simulink model "FaultCheck"  (R2022b)
settings: Solver=FixedStepAuto  StartTime=0.0  StopTime=10  FixedStep=1  RelTol=1e-3
undefined symbols (not defined in the file): C_Flt_IGBTULowerTempConfirmTh_u16, C_Flt_IGBTULowerTempDiagEn_b, C_Flt_IGBTULowerTempErrCode_u16, C_Flt_IGBTULowerTempPowerCoeff, C_Flt_IGBTULowerTempRecoveryTh_u16, C_Flt_IGBTULowerTempRecTh_s32, C_Flt_IGBTULowerTempTrigTh_s32, C_Flt_IGBTUOverTempConfirmTh_u16, C_Flt_IGBTUOverTempDiagEn_b, C_Flt_IGBTUOverTempErrCode_u16, C_Flt_IGBTUOverTempRecoveryTh_u16, C_Flt_IGBTUOverTempRecTh_s32, C_Flt_IGBTUOverTempTrigTh_s32, C_Flt_IGBTVLowerTempConfirmTh_u16, C_Flt_IGBTVLowerTempDiagEn_b, C_Flt_IGBTVLowerTempErrCode_u16, C_Flt_IGBTVLowerTempPowerCoeff, C_Flt_IGBTVLowerTempRecoveryTh_u16, C_Flt_IGBTVLowerTempRecTh_s32, C_Flt_IGBTVLowerTempTrigTh_s32, C_Flt_IGBTVOverTempConfirmTh_u16, C_Flt_IGBTVOverTempDiagEn_b, C_Flt_IGBTVOverTempErrCode_u16, C_Flt_IGBTVOverTempRecoveryTh_u16, C_Flt_IGBTVOverTempRecTh_s32, C_Flt_IGBTVOverTempTrigTh_s32, C_Flt_IGBTWLowerTempConfirmTh_u16, C_Flt_IGBTWLowerTempDiagEn_b, C_Flt_IGBTWLowerTempErrCode_u16, C_Flt_IGBTWLowerTempPowerCoeff, C_Flt_IGBTWLowerTempRecoveryTh_u16, C_Flt_IGBTWLowerTempRecTh_s32, C_Flt_IGBTWLowerTempTrigTh_s32, C_Flt_IGBTWOverTempConfirmTh_u16, C_Flt_IGBTWOverTempDiagEn_b, C_Flt_IGBTWOverTempErrCode_u16, C_Flt_IGBTWOverTempRecoveryTh_u16, C_Flt_IGBTWOverTempRecTh_s32, C_Flt_IGBTWOverTempTrigTh_s32, C_Flt_IuOCConfirmTh_u16, C_Flt_IuOCDiagEn_b, C_Flt_IuOCErrCode_u16, C_Flt_IuOCNegLimit_s32, C_Flt_IuOCPosLimit_s32, C_Flt_IuOCRecoveryTh_u16, C_Flt_IuZeroDriftDiagEn_b, C_Flt_IuZeroDriftErrCode_u16, C_Flt_IvOCConfirmTh_u16, C_Flt_IvOCDiagEn_b, C_Flt_IvOCErrCode_u16, C_Flt_IvOCNegLimit_s32, C_Flt_IvOCPosLimit_s32, C_Flt_IvOCRecoveryTh_u16, C_Flt_IvZeroDriftDiagEn_b, C_Flt_IvZeroDriftErrCode_u16, C_Flt_IwOCConfirmTh_u16, C_Flt_IwOCDiagEn_b, C_Flt_IwOCErrCode_u16, C_Flt_IwOCNegLimit_s32, C_Flt_IwOCPosLimit_s32 ... (+196)
libraries: YS_UserDefined_Library x21, simulink x5
(part 2 of 11)

== system FaultCheck/FaultDiag_HighTask_100us/FltDetn/RecUDetn ==
  note: Flt_RecU_ErrDeb
      | Uint8
      | 旋变电压故障判断次数
      |
      | Flt_RecU_ActvnErrDetn
      | Uint8
      | 旋变电压故障使能标志位
      |
      | Flt_RecU_ErrCode
      | Uint16
      | 旋变电压故障码
  note: 故障诊断主体模块主要包括四个部分，故障诊断标志位判断、故障等级判断、降功率系数判断和故障码记录
      | 1、故障诊断标志位判断：根据使能标志位判断进入，最后确认其故障标志位的值
      | 2、故障码记录：根据故障标志位记录相关故障码，0还是标定量。
      | 3、故障等级判断：根据故障标志位确定相关故障等级，是0还是标定量
      | 4、降功率系数判断：根据故障等级进行判断选择对应的降功率系数
      |
      | 故障标志位的判断：
      | 当输入的旋变供电标志位标志位为1，并持续标定的次数，故障标志位置1，否者保留上一时刻的故障标志位0，不可恢复。
  IPT_Res_Udc_Error_Flg : Inport
  Sys_SelfChkFishFlg : Inport  Port=2
  Bus Creator : BusCreator  Inputs=2
  Enable : Subsystem
  Parameter : Subsystem
  RecUDetn : Subsystem
  Flt_RecUDetnOut : Outport
  wires:
  Sys_SelfChkFishFlg/1 -> Enable/1(Sys_SelfChkFishFlg)
  Enable/1(Enable) -> RecUDetn/2(EnabDetn)
  RecUDetn/1(Flt_RecUFltLvl) -> Bus Creator/1
  RecUDetn/2(Flt_RecUPowRecCoefOut) -> Bus Creator/2
  Parameter/1(Para) -> RecUDetn/3(Para)
  Bus Creator/1 -> Flt_RecUDetnOut/1
  IPT_Res_Udc_Error_Flg/1 -> RecUDetn/1(InPutVal)

== system FaultCheck/FaultDiag_HighTask_100us/FltDetn/ResErrFlgDetn ==
  note: Flt_ResErr_ActvnDetn
      | Uint8
      | 旋变信号故障判断次数
      |
      | Flt_ResErr_ErrCode
      | Uint16
      | 旋变信号故障码
  note: 故障诊断主体模块主要包括四个部分，故障诊断标志位判断、故障等级判断、降功率系数判断和故障码记录
      | 1、故障诊断标志位判断：根据使能标志位判断进入，最后确认其故障标志位的值
      | 2、故障码记录：根据故障标志位记录相关故障码，0还是标定量。
      | 3、故障等级判断：根据故障标志位确定相关故障等级，是0还是标定量
      | 4、降功率系数判断：根据故障等级进行判断选择对应的降功率系数
      |
      | 故障标志位的判断：
      | 当输入的旋变信号故障标志位标志位为1，并持续标定的次数，故障标志位置1，否者保留上一时刻的故障标志位0，不可恢复。
  IPT_Hw_RES_LOT_Error_Flg : Inport
  IPT_Hw_RES_LOS_Error_Flg : Inport  Port=2
  Sys_SelfChkFishFlg : Inport  Port=3
  Bus Creator : BusCreator  Inputs=2
  Enable : Subsystem
  Logical Operator : Logic  Operator=OR  AllPortsSameDT=off  OutDataTypeStr=boolean
  Parameter : Subsystem
  ResErrDetn : Subsystem
  Flt_ResErrFlgDetnOut : Outport
  wires:
  Enable/1(Enable) -> ResErrDetn/2(EnabDetn)
  ResErrDetn/1(Flt_ResErrFltLvl) -> Bus Creator/1
  ResErrDetn/2(Flt_ResErrPowRecCoefOut) -> Bus Creator/2
  Parameter/1(Para) -> ResErrDetn/3(Para)
  Bus Creator/1 -> Flt_ResErrFlgDetnOut/1
  Sys_SelfChkFishFlg/1 -> Enable/1(Sys_SelfChkFishFlg)
  IPT_Hw_RES_LOT_Error_Flg/1 -> Logical Operator/1
  IPT_Hw_RES_LOS_Error_Flg/1 -> Logical Operator/2
  Logical Operator/1 -> ResErrDetn/1(InPutVal1)

== system FaultCheck/FaultDiag_HighTask_100us/FltDetn/ResolveSensorDetn ==
  Sys_SelfChkFishFlg : Inport
  Flt_ResolveSensorFlg : Inport  Port=2
  Bus Creator : BusCreator  Inputs=2
  Enable : Subsystem
  Flt_ResolveSensorDetn : Subsystem
  Parameter : Subsystem
  Flt_ResolveSensorDetnOut : Outport
  wires:
  Parameter/1(Para) -> Flt_ResolveSensorDetn/3(Para)
  Enable/1(Enable) -> Flt_ResolveSensorDetn/2(EnabDetn)
  Bus Creator/1 -> Flt_ResolveSensorDetnOut/1
  Sys_SelfChkFishFlg/1 -> Enable/1(Sys_SelfChkFishFlg)
  Flt_ResolveSensorDetn/2(Flt_ResolveSensorPowRecCoefOut) -> Bus Creator/2
  Flt_ResolveSensorDetn/1(Flt_ResolveSensorFltLvl) -> Bus Creator/1
  Flt_ResolveSensorFlg/1 -> Flt_ResolveSensorDetn/1(InPutVal1)

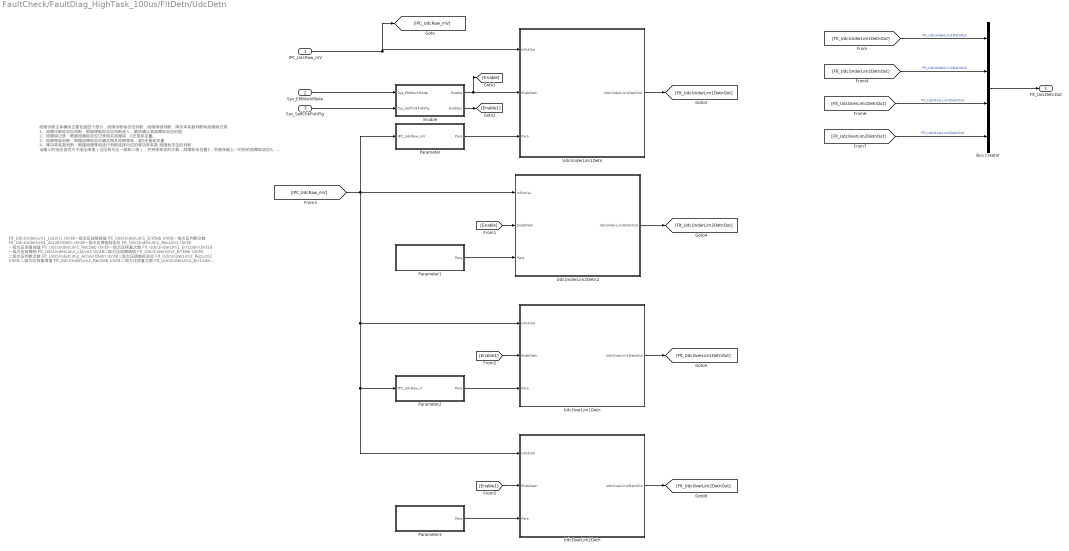
== system FaultCheck/FaultDiag_HighTask_100us/FltDetn/UdcDetn ==
  note: Flt_UdcUnderLim1_LoLim1
      | Uint8
      | 一级欠压故障阈值
      |
      | Flt_UdcUnderLim1_ErrDeb
      | Uint8
      | 一级欠压判断次数
      |
      | Flt_UdcUnderLim1_ActvErrDetn
      | Uint8
      | 一级欠压使能标志位
      |
      | Flt_UdcUnderLim1_RecLim1
      | Uint8
      | 一级欠压恢复阈值
      |
      | Flt_UdcUnderLim1_RecDeb
      | Uint8
      | 一级欠压恢复次数
      |
      | Flt_UdcUnderLim1_ErrCode
      | Uint16
      | 一级欠压故障码
      |
      | Flt_UdcUnderLim2_LoLim2
      | Uint8
      | 二级欠压故障阈值
      |
      | Flt_UdcUnderLim2_ErrDeb
      | Uint8
      | 二级欠压判断次数
      |
      | Flt_UdcUnderLim2_ActvErrDetn
      | Uint8
      | 二级欠压使能标志位
      |
      | Flt_UdcUnderLim2_RecLim2
      | Uint8
      | 二级欠压恢复阈值
      |
      | Flt_UdcUnderLim2_RecDeb
      | Uint8
      | 二级欠压恢复次数
      |
      | Flt_UdcUnderLim2_ErrCode
      | Uint16
      | 二级欠压故障码
      |
      | Flt_UdcOverLim1_OverLim1
      | Uint8
      | 一级过压故障阈值
      |
      | Flt_UdcOverLim1_ErrDeb
      | Uint8
      | 一级过压判断次数
      |
      | Flt_UdcOverLim1_ActvErrDetn
      | Uint8
      | 一级过压使能标志位
      |
      | Flt_UdcOverLim1_RecLim1
      | Uint8
      | 一级过压恢复阈值
      |
      | Flt_UdcOverLim1_RecDeb
      | Uint8
      | 一级过压恢复次数
      |
      | Flt_UdcOverLim1_ErrCode
      | Uint16
      | 一级过压故障码
      |
      | Flt_UdcOverLim2_OverLim2
      | Uint8
      | 二过压故障阈值
      |
      | Flt_UdcOverLim2_ErrDeb
      | Uint8
      | 二级过压判断次数
      |
      | Flt_UdcOverLim2_ActvErrDetn
      | Uint8
      | 二级过压使能标志位
      |
      | Flt_UdcOverLim2_ErrCode
      | Uint16
      | 二级过压故障码
  note: 故障诊断主体模块主要包括四个部分，故障诊断标志位判断、故障等级判断、降功率系数判断和故障码记录
      | 1、故障诊断标志位判断：根据使能标志位判断进入，最后确认其故障标志位的值
      | 2、故障码记录：根据故障标志位记录相关故障码，0还是标定量。
      | 3、故障等级判断：根据故障标志位确定相关故障等级，是0还是标定量
      | 4、降功率系数判断：根据故障等级进行判断选择对应的降功率系数
      |
      | 故障标志位的判断：
      | 当输入的电压信号大于电压阈值（过压和欠压一级和二级），并持续标定的次数，故障标志位置1，否者保留上一时刻的故障标志位0。
      |
      | 一级和二级欠压，一级过压可恢复，即当输入的电压信号小于恢复的阈值并持续标定的次数，故障标志位置0
      |
      | 二级过压不可恢复
  IPC_UdcRaw_mV : Inport
  Sys_EMWorkMode : Inport  Port=2
  Sys_SelfChkFishFlg : Inport  Port=3
  Bus Creator : BusCreator  Inputs=4
  Enable : Subsystem
  Parameter : Subsystem
  Parameter1 : Subsystem
  Parameter2 : Subsystem
  Parameter3 : Subsystem
  UdcOverLim1Detn : Subsystem
  UdcOverLim2Detn : Subsystem
  UdcUnderLim1Detn : Subsystem
  UdcUnderLim2Detn2 : Subsystem
  Flt_UdcDetnOut : Outport
  wires:
  [IPC_UdcRaw_mV] -> UdcUnderLim2Detn2/1(InPutVal), Parameter/1(IPC_UdcRaw_mV), UdcOverLim2Detn/1(InPutVal), Parameter2/1(IPC_UdcRaw_V), UdcOverLim1Detn/1(InPutVal)
  [Flt_UdcOverLim2DetnOut] -> Bus Creator/4  "Flt_UdcOverLim2DetnOut"
  [Flt_UdcOverLim1DetnOut] -> Bus Creator/3  "Flt_UdcOverLim1DetnOut"
  [Flt_UdcUnderLim2DetnOut] -> Bus Creator/2  "Flt_UdcUnderLim2DetnOut"
  [Flt_UdcUnderLim1DetnOut] -> Bus Creator/1  "Flt_UdcUnderLim1DetnOut"
  UdcOverLim2Detn/1(UdcOverLim2DetnOut) -> [Flt_UdcOverLim2DetnOut]
  UdcOverLim1Detn/1(UdcOverLim1DetnOut) -> [Flt_UdcOverLim1DetnOut]
  UdcUnderLim2Detn2/1(UdcUnderLim2DetnOut) -> [Flt_UdcUnderLim2DetnOut]
  UdcUnderLim1Detn/1(UdcUnderLim1DetnOut) -> [Flt_UdcUnderLim1DetnOut]
  [Enable1] -> UdcOverLim2Detn/2(EnabDetn)
  Parameter3/1(Para) -> UdcOverLim2Detn/3(Para)
  Enable/2(Enable1) -> [Enable1]
  Parameter2/1(Para) -> UdcOverLim1Detn/3(Para)
  [Enable1] -> UdcOverLim1Detn/2(EnabDetn)
  Parameter1/1(Para) -> UdcUnderLim2Detn2/3(Para)
  [Enable] -> UdcUnderLim2Detn2/2(EnabDetn)
  Sys_SelfChkFishFlg/1 -> Enable/2(Sys_SelfChkFishFlg)
  Bus Creator/1 -> Flt_UdcDetnOut/1
  Sys_EMWorkMode/1 -> Enable/1(Sys_EMWorkMode)
  Enable/1(Enable) -> UdcUnderLim1Detn/2(EnabDetn), [Enable]
  Parameter/1(Para) -> UdcUnderLim1Detn/3(Para)
  IPC_UdcRaw_mV/1 -> [IPC_UdcRaw_mV], UdcUnderLim1Detn/1(InPutVal)

== system FaultCheck/FaultDiag_HighTask_100us/FltDetn/UdcZeroDrfDetn ==
  CurrentReadingCaliFlag : Inport
  Trigger : TriggerPort  VariantControl=(inherit)  PortDimensions=1
  Bus Creator : BusCreator  Inputs=2
  Enable : Subsystem
  Parameter : Subsystem
  UdcZeroDrfDetn : Subsystem
  Flt_UdcZeroDrfDetn : Outport
  wires:
  CurrentReadingCaliFlag/1 -> UdcZeroDrfDetn/1(InPutVal)
  Enable/1(Enable) -> UdcZeroDrfDetn/2(EnabDetn)
  Bus Creator/1 -> Flt_UdcZeroDrfDetn/1
  UdcZeroDrfDetn/2(Flt_UdcZeroDrfPowRecCoefOut) -> Bus Creator/2
  Parameter/1(Para) -> UdcZeroDrfDetn/3(Para)
  UdcZeroDrfDetn/1(Flt_UdcZeroDrfFltLvl) -> Bus Creator/1

== system FaultCheck/FaultDiag_HighTask_100us/FltDetn/VoltagSensorDetn ==
  Sys_SelfChkFishFlg : Inport
  Flt_VoltagSensorFlg : Inport  Port=2
  IPT_UdcRaw_mV : Inport  Port=3
  Bus Creator : BusCreator  Inputs=2
  Enable : Subsystem
  Flt_VoltagSensorDetn : Subsystem
  Parameter : Subsystem
  Flt_VoltagSensorDetnOut : Outport
  wires:
  Sys_SelfChkFishFlg/1 -> Enable/1(Sys_SelfChkFishFlg)
  Flt_VoltagSensorDetn/2(Flt_VoltagSensorPowRecCoefOut) -> Bus Creator/2
  IPT_UdcRaw_mV/1 -> Flt_VoltagSensorDetn/4(IPT_UdcRaw_mV)
  Bus Creator/1 -> Flt_VoltagSensorDetnOut/1
  Flt_VoltagSensorDetn/1(Flt_VoltagSensorFltLvl) -> Bus Creator/1
  Parameter/1(Para) -> Flt_VoltagSensorDetn/3(Para)
  Enable/1(Enable) -> Flt_VoltagSensorDetn/2(EnabDetn)
  Flt_VoltagSensorFlg/1 -> Flt_VoltagSensorDetn/1(InPutVal1)

== system FaultCheck/FaultDiag_HighTask_100us/FltHandle/FltLvl ==
  FltDetnIn : Inport
  Bus Selector : BusSelector  OutputSignals=Flt_OverCurrDetnOut.Flt_IuOverCurrDetnOut.Flt_IuOverCurrFltLvlOut,Flt_OverCurrDetnOut.Flt_IvOverCurrDetnOut.Flt_IvOverCurrFltLvlOut,Flt_OverCurrDetnOut.Flt_IwOverCurrDetnOut.Flt_IwOverCurrFltLvlOut,Flt_HWOverCurrDetnOut.Flt_HWOverCurrFltLvl,Flt_Drive_L_DetnOut.Flt_Drive_L_FltLvl,Flt_Drive_H_DetnOut.Flt_Drive_H_FltLvl,Flt_DriveUdcDetnOut.Flt_DriveUdcFltLvl,Flt_HWOverUdcDetnOut.Flt_HWOverUdcFltLvl,Flt_CurrZeroDrfDetnOut.Flt_CurrZeroDrfFltLv,Flt_ResErrFlgDetnOut.Flt_ResErrFltLvl,Flt_UdcDetnOut.Flt_UdcUnderLim1DetnOut.Flt_UdcUnderLim1FltLvlOut,Flt_UdcDetnOut.Flt_UdcUnderLim2DetnOut.Flt_UdcUnderLim2FltLvlOut,Flt_UdcDetnOut.Flt_UdcOverLim1DetnOut.Flt_UdcOverLim1FltLvlOut,Flt_UdcDetnOut.Flt_UdcOverLim2DetnOut.Flt_UdcOverLim2FltLvlOut,Flt_RecUDetnOut.Flt_RecUFltLvl
  Min of Elements : MinMax  Function=max  Inputs=15
  Flt_HighTaskFltLvlOut : Outport
  wires:
  Min of Elements/1 -> Flt_HighTaskFltLvlOut/1
  FltDetnIn/1 -> Bus Selector/1
  Bus Selector/1 -> Min of Elements/1  "<Flt_IuOverCurrFltLvlOut>"
  Bus Selector/2 -> Min of Elements/2  "<Flt_IvOverCurrFltLvlOut>"
  Bus Selector/3 -> Min of Elements/3  "<Flt_IwOverCurrFltLvlOut>"
  Bus Selector/4 -> Min of Elements/4  "<Flt_HWOverCurrFltLvl>"
  Bus Selector/5 -> Min of Elements/5  "<Flt_Drive_L_FltLvl>"
  Bus Selector/6 -> Min of Elements/6  "<Flt_Drive_H_FltLvl>"
  Bus Selector/7 -> Min of Elements/7  "<Flt_DriveUdcFltLvl>"
  Bus Selector/8 -> Min of Elements/8  "<Flt_HWOverUdcFltLvl>"
  Bus Selector/9 -> Min of Elements/9  "<Flt_CurrZeroDrfFltLv>"
  Bus Selector/10 -> Min of Elements/10  "<Flt_ResErrFltLvl>"
  Bus Selector/11 -> Min of Elements/11  "<Flt_UdcUnderLim1FltLvlOut>"
  Bus Selector/12 -> Min of Elements/12  "<Flt_UdcUnderLim2FltLvlOut>"
  Bus Selector/13 -> Min of Elements/13  "<Flt_UdcOverLim1FltLvlOut>"
  Bus Selector/14 -> Min of Elements/14  "<Flt_UdcOverLim2FltLvlOut>"
  Bus Selector/15 -> Min of Elements/15  "<Flt_RecUFltLvl>"

== system FaultCheck/FaultDiag_HighTask_100us/FltHandle/PowRecCoef ==
  FltDetnIn : Inport
  Bus Selector : BusSelector  OutputSignals=Flt_OverCurrDetnOut.Flt_IuOverCurrDetnOut.Flt_IuOverCurrPowRecCoefOut,Flt_Drive_L_DetnOut.Flt_Drive_L_PowRecCoefOut,Flt_Drive_H_DetnOut.Flt_Drive_H_PowRecCoefOut,Flt_DriveUdcDetnOut.Flt_DriveUdcPowRecCoefOut,Flt_HWOverUdcDetnOut.Flt_HWOverUdcPowRecCoefOut,Flt_OverCurrDetnOut.Flt_IvOverCurrDetnOut.Flt_IvOverCurrPowRecCoefOut,Flt_OverCurrDetnOut.Flt_IwOverCurrDetnOut.Flt_IwOverCurrPowRecCoefOut,Flt_HWOverCurrDetnOut.Flt_HWOverCurrPowRecCoefOut,Flt_CurrZeroDrfDetnOut.Flt_CurrZeroDrfPowRecCoefOut,Flt_ResErrFlgDetnOut.Flt_ResErrPowRecCoefOut,Flt_UdcDetnOut.Flt_UdcUnderLim1DetnOut.Flt_UdcUnderLim1RecCoefOut,Flt_UdcDetnOut.Flt_UdcUnderLim2DetnOut.Flt_UdcUnderLim2RecCoefOut,Flt_UdcDetnOut.Flt_UdcOverLim1DetnOut.Flt_UdcOverLim1RecCoefOut,Flt_UdcDetnOut.Flt_UdcOverLim2DetnOut.Flt_UdcOverLim2RecCoefOut,Flt_RecUDetnOut.Flt_RecUPowRecCoefOut
  Min of Elements : MinMax  Inputs=15
  Flt_HighTaskPowRecCoef : Outport
  wires:
  FltDetnIn/1 -> Bus Selector/1
  Min of Elements/1 -> Flt_HighTaskPowRecCoef/1
  Bus Selector/1 -> Min of Elements/1  "<Flt_IuOverCurrPowRecCoefOut>"
  Bus Selector/2 -> Min of Elements/2  "<Flt_Drive_L_PowRecCoefOut>"
  Bus Selector/3 -> Min of Elements/3  "<Flt_Drive_H_PowRecCoefOut>"
  Bus Selector/4 -> Min of Elements/4  "<Flt_DriveUdcPowRecCoefOut>"
  Bus Selector/5 -> Min of Elements/5  "<Flt_HWOverUdcPowRecCoefOut>"
  Bus Selector/6 -> Min of Elements/6  "<Flt_IvOverCurrPowRecCoefOut>"
  Bus Selector/7 -> Min of Elements/7  "<Flt_IwOverCurrPowRecCoefOut>"
  Bus Selector/8 -> Min of Elements/8  "<Flt_HWOverCurrPowRecCoefOut>"
  Bus Selector/9 -> Min of Elements/9  "<Flt_CurrZeroDrfPowRecCoefOut>"
  Bus Selector/10 -> Min of Elements/10  "<Flt_ResErrPowRecCoefOut>"
  Bus Selector/11 -> Min of Elements/11  "<Flt_UdcUnderLim1RecCoefOut>"
  Bus Selector/12 -> Min of Elements/12  "<Flt_UdcUnderLim2RecCoefOut>"
  Bus Selector/13 -> Min of Elements/13  "<Flt_UdcOverLim1RecCoefOut>"
  Bus Selector/14 -> Min of Elements/14  "<Flt_UdcOverLim2RecCoefOut>"
  Bus Selector/15 -> Min of Elements/15  "<Flt_RecUPowRecCoefOut>"

== system FaultCheck/FaultDiag_HighTask_100us/FltHandle/ValOut ==
  FltSignalBus : Inport
  CurrentVal : Subsystem
  Flt_IuOut_A : Outport
  Flt_IvOut_A : Outport  Port=2
  Flt_IwOut_A : Outport  Port=3
  wires:
  CurrentVal/1(Flt_IuOut_A) -> Flt_IuOut_A/1
  FltSignalBus/1 -> CurrentVal/1(FltSignalBus)
  CurrentVal/2(Flt_IvOut_A) -> Flt_IvOut_A/1
  CurrentVal/3(Flt_IwOut_A1) -> Flt_IwOut_A/1

== system FaultCheck/FaultDiagnose/CurrZeroDriftFltDiag/IuZeroDriftDiag ==
  SysSelfCheckDownFlg : Inport
  IuZeroDriftFltFlg : Inport  Port=2
  Enable : EnablePort
  Bus Creator : BusCreator  Inputs=3
  Bus Selector : BusSelector  OutputSignals=IuZeroDriftDiagEn
  Bus Selector1 : BusSelector  OutputSignals=IuZeroDriftFltLevel
  Bus Selector2 : BusSelector  OutputSignals=IuZeroDriftPowerCoeff
  Constant : Constant  OutDataTypeStr=boolean
  Diagnose : Subsystem
  FaultLevelDeter : Subsystem
  Parameters : Subsystem
  PowerReductionCoeffDeter : Subsystem
  Unit Delay : UnitDelay  SampleTime=-1  HasFrameUpgradeWarning=on
  IuZeroDriftDiagDownFlg : Outport
  IuZeroDriftFltInfo : Outport  Port=2
  wires:
  Constant/1 -> Unit Delay/1
  Unit Delay/1 -> IuZeroDriftDiagDownFlg/1
  Parameters/1(IuZeroDriftParam) -> Bus Selector/1, Bus Selector2/1, Bus Selector1/1
  Bus Selector/1 -> Diagnose/1(IuZeroDftEn)  "<IuZeroDriftDiagEn>"
  IuZeroDriftFltFlg/1 -> Diagnose/2(IuZeroDriftFltFlg)
  Bus Selector2/1 -> PowerReductionCoeffDeter/2(PowerCoeff)  "<IuZeroDriftPowerCoeff>"
  Diagnose/1(IuZeroDriftFltFlgOut) -> Bus Creator/1, FaultLevelDeter/1(IuZeroDriftFltFlgOut)
  Bus Selector1/1 -> FaultLevelDeter/2(FaultLevel)  "<IuZeroDriftFltLevel>"
  FaultLevelDeter/1(IuZeroDriftFltLevelOut) -> PowerReductionCoeffDeter/1(IuZeroDriftFltLevelOut), Bus Creator/2
  PowerReductionCoeffDeter/1(IuZeroDriftPowerCoeff) -> Bus Creator/3
  Bus Creator/1 -> IuZeroDriftFltInfo/1
  SysSelfCheckDownFlg/1 -> Diagnose/3(SysSelfCheckDownFlg)

== system FaultCheck/FaultDiagnose/CurrZeroDriftFltDiag/IvZeroDriftDiag ==
  SysSelfCheckDownFlg : Inport
  IvZeroDriftFltFlg : Inport  Port=2
  Enable : EnablePort
  Bus Creator : BusCreator  Inputs=3
  Bus Selector : BusSelector  OutputSignals=IvZeroDriftDiagEn
  Bus Selector1 : BusSelector  OutputSignals=IvZeroDriftFltLevel
  Bus Selector2 : BusSelector  OutputSignals=IvZeroDriftPowerCoeff
  Constant : Constant  OutDataTypeStr=boolean
  Diagnose : Subsystem
  FaultLevelDeter : Subsystem
  Parameters : Subsystem
  PowerReductionCoeffDeter : Subsystem
  Unit Delay : UnitDelay  SampleTime=-1  HasFrameUpgradeWarning=on
  IvZeroDriftDiagDownFlg : Outport
  IvZeroDriftFltInfo : Outport  Port=2
  wires:
  Bus Creator/1 -> IvZeroDriftFltInfo/1
  PowerReductionCoeffDeter/1(IvZeroDriftPowerCoeff) -> Bus Creator/3
  FaultLevelDeter/1(IvZeroDriftFltLevelOut) -> Bus Creator/2, PowerReductionCoeffDeter/1(IvZeroDriftFltLevelOut)
  Bus Selector1/1 -> FaultLevelDeter/2(FaultLevel)  "<IvZeroDriftFltLevel>"
  Diagnose/1(IvZeroDriftFltFlgOut) -> FaultLevelDeter/1(IvZeroDriftFltFlgOut), Bus Creator/1
  Bus Selector2/1 -> PowerReductionCoeffDeter/2(PowerCoeff)  "<IvZeroDriftPowerCoeff>"
  IvZeroDriftFltFlg/1 -> Diagnose/2(IvZeroDriftFltFlg)
  Bus Selector/1 -> Diagnose/1(IvZeroDftEn)  "<IvZeroDriftDiagEn>"
  Parameters/1(IvZeroDriftParam) -> Bus Selector1/1, Bus Selector2/1, Bus Selector/1
  Unit Delay/1 -> IvZeroDriftDiagDownFlg/1
  Constant/1 -> Unit Delay/1
  SysSelfCheckDownFlg/1 -> Diagnose/3(SysSelfCheckDownFlg)

== system FaultCheck/FaultDiagnose/CurrZeroDriftFltDiag/IwZeroDriftDiag ==
  SysSelfCheckDownFlg : Inport
  IwZeroDriftFltFlg : Inport  Port=2
  Enable : EnablePort
  Bus Creator : BusCreator  Inputs=3
  Bus Selector : BusSelector  OutputSignals=IwZeroDriftDiagEn
  Bus Selector1 : BusSelector  OutputSignals=IwZeroDriftFltLevel
  Bus Selector2 : BusSelector  OutputSignals=IwZeroDriftPowerCoeff
  Constant : Constant  OutDataTypeStr=boolean
  Diagnose : Subsystem
  FaultLevelDeter : Subsystem
  Parameters : Subsystem
  PowerReductionCoeffDeter : Subsystem
  Unit Delay : UnitDelay  SampleTime=-1  HasFrameUpgradeWarning=on
  IwZeroDriftDiagDownFlg : Outport
  IwZeroDriftFltInfo : Outport  Port=2
  wires:
  Constant/1 -> Unit Delay/1
  Unit Delay/1 -> IwZeroDriftDiagDownFlg/1
  Parameters/1(IwZeroDriftParam) -> Bus Selector/1, Bus Selector2/1, Bus Selector1/1
  Bus Selector/1 -> Diagnose/1(IwZeroDftEn)  "<IwZeroDriftDiagEn>"
  IwZeroDriftFltFlg/1 -> Diagnose/2(IwZeroDriftFltFlg)
  Bus Selector2/1 -> PowerReductionCoeffDeter/2(PowerCoeff)  "<IwZeroDriftPowerCoeff>"
  Diagnose/1(IwZeroDriftFltFlgOut) -> FaultLevelDeter/1(IwZeroDriftFltFlgOut), Bus Creator/1
  Bus Selector1/1 -> FaultLevelDeter/2(FaultLevel)  "<IwZeroDriftFltLevel>"
  FaultLevelDeter/1(IwZeroDriftFltLevelOut) -> PowerReductionCoeffDeter/1(IwZeroDriftFltLevelOut), Bus Creator/2
  PowerReductionCoeffDeter/1(IwZeroDriftPowerCoeff) -> Bus Creator/3
  Bus Creator/1 -> IwZeroDriftFltInfo/1
  SysSelfCheckDownFlg/1 -> Diagnose/3(SysSelfCheckDownFlg)

== system FaultCheck/FaultDiagnose/IGBTTempDiag/IGBTULowerTempDiag ==
  SysSelfCheckDownFlg : Inport
  IGBTUTemp : Inport  Port=2
  Bus Creator : BusCreator  Inputs=3
  Bus Selector : BusSelector  OutputSignals=IGBTULowerTempDiagEn
  Bus Selector1 : BusSelector  OutputSignals=IGBTULowerTempFltLevel,IGBTULowerTempPowerCoeff
  Diagnose : Subsystem
  EnableJudgement : Subsystem
  FaultLevelDeter : Subsystem
  Parameters : Subsystem
  PowerReductionCoeffDeter : Subsystem
  IGBTULowerTempFltInfo : Outport
  wires:
  Bus Selector/1 -> EnableJudgement/2(DiagEn)  "<IGBTULowerTempDiagEn>"
  Bus Selector1/2 -> PowerReductionCoeffDeter/2(PowerCoeff)  "<IGBTULowerTempPowerCoeff>"
  IGBTUTemp/1 -> Diagnose/2(IGBTUTemp)
  PowerReductionCoeffDeter/1(IGBTULowerTempPowerCoeffOut) -> Bus Creator/3  "IGBTULowerTempPowerCoeffOut"
  FaultLevelDeter/1(IGBTULowerTempFltLevelOut) -> PowerReductionCoeffDeter/1(IGBTULowerTempFltLevelOut), Bus Creator/2  "IGBTULowerTempFltLevelOut"
  Diagnose/1(IGBTULowerTempFlgOut) -> FaultLevelDeter/1(IGBTULowerTempFlgOut), Bus Creator/1  "IGBTULowerTempFlgOut"
  EnableJudgement/1(DiagEnOut) -> Diagnose/1(DiagEnOut)
  SysSelfCheckDownFlg/1 -> EnableJudgement/1(SysSelfCheckDownFlg)
  Parameters/1(Param) -> Bus Selector/1, Diagnose/3(Parameter), Bus Selector1/1
  Bus Creator/1 -> IGBTULowerTempFltInfo/1
  Bus Selector1/1 -> FaultLevelDeter/2(FaultLevel)  "<IGBTULowerTempFltLevel>"

== system FaultCheck/FaultDiagnose/IGBTTempDiag/IGBTUOverTempDiag ==
  SysSelfCheckDownFlg : Inport
  IGBTUTemp : Inport  Port=2
  Bus Creator : BusCreator  Inputs=3
  Bus Selector : BusSelector  OutputSignals=IGBTUOverTempDiagEn
  Bus Selector1 : BusSelector  OutputSignals=IGBTUOverTempFltLevel,IGBTUOverTempPowerCoeff
  Diagnose : Subsystem
  EnableJudgement : Subsystem
  FaultLevelDeter : Subsystem
  Parameters : Subsystem
  PowerReductionCoeffDeter : Subsystem
  IGBTUOverTempFltInfo : Outport
  wires:
  Bus Selector1/1 -> FaultLevelDeter/2(FaultLevel)  "<IGBTUOverTempFltLevel>"
  Bus Creator/1 -> IGBTUOverTempFltInfo/1
  Parameters/1(Param) -> Bus Selector1/1, Diagnose/3(Parameter), Bus Selector/1
  SysSelfCheckDownFlg/1 -> EnableJudgement/1(SysSelfCheckDownFlg)
  EnableJudgement/1(DiagEnOut) -> Diagnose/1(DiagEnOut)
  Diagnose/1(IGBTUOverTempFlgOut) -> Bus Creator/1, FaultLevelDeter/1(IGBTUOverTempFlgOut)  "IGBTUOverTempFlgOut"
  FaultLevelDeter/1(IGBTUOverTempFltLevelOut) -> Bus Creator/2, PowerReductionCoeffDeter/1(IGBTUOverTempFltLevelOut)  "IGBTUOverTempFltLevelOut"
  PowerReductionCoeffDeter/1(IGBTUOverTempPowerCoeffOut) -> Bus Creator/3  "IGBTUOverTempPowerCoeffOut"
  IGBTUTemp/1 -> Parameters/1(IGBTUTemp), Diagnose/2(IGBTUTemp)
  Bus Selector1/2 -> PowerReductionCoeffDeter/2(PowerCoeff)  "<IGBTUOverTempPowerCoeff>"
  Bus Selector/1 -> EnableJudgement/2(DiagEn)  "<IGBTUOverTempDiagEn>"

== system FaultCheck/FaultDiagnose/IGBTTempDiag/IGBTVLowerTempDiag ==
  SysSelfCheckDownFlg : Inport
  IGBTVTemp : Inport  Port=2
  Bus Creator : BusCreator  Inputs=3
  Bus Selector : BusSelector  OutputSignals=IGBTVLowerTempDiagEn
  Bus Selector1 : BusSelector  OutputSignals=IGBTVLowerTempFltLevel,IGBTVLowerTempPowerCoeff
  Diagnose : Subsystem
  EnableJudgement : Subsystem
  FaultLevelDeter : Subsystem
  Parameters : Subsystem
  PowerReductionCoeffDeter : Subsystem
  IGBTVLowerTempFltInfo : Outport
  wires:
  Bus Selector1/1 -> FaultLevelDeter/2(FaultLevel)  "<IGBTVLowerTempFltLevel>"
  Bus Creator/1 -> IGBTVLowerTempFltInfo/1
  Parameters/1(Param) -> Bus Selector1/1, Diagnose/3(Parameter), Bus Selector/1
  SysSelfCheckDownFlg/1 -> EnableJudgement/1(SysSelfCheckDownFlg)
  EnableJudgement/1(DiagEnOut) -> Diagnose/1(DiagEnOut)
  Diagnose/1(IGBTVLowerTempFlgOut) -> Bus Creator/1, FaultLevelDeter/1(IGBTVLowerTempFlgOut)  "IGBTVLowerTempFlgOut"
  FaultLevelDeter/1(IGBTVLowerTempFltLevelOut) -> Bus Creator/2, PowerReductionCoeffDeter/1(IGBTVLowerTempFltLevelOut)  "IGBTVLowerTempFltLevelOut"
  PowerReductionCoeffDeter/1(IGBTVLowerTempPowerCoeffOut) -> Bus Creator/3  "IGBTVLowerTempPowerCoeffOut"
  IGBTVTemp/1 -> Diagnose/2(IGBTVTemp)
  Bus Selector1/2 -> PowerReductionCoeffDeter/2(PowerCoeff)  "<IGBTVLowerTempPowerCoeff>"
  Bus Selector/1 -> EnableJudgement/2(DiagEn)  "<IGBTVLowerTempDiagEn>"

== system FaultCheck/FaultDiagnose/IGBTTempDiag/IGBTVOverTempDiag ==
  SysSelfCheckDownFlg : Inport
  IGBTVTemp : Inport  Port=2
  Bus Creator : BusCreator  Inputs=3
  Bus Selector : BusSelector  OutputSignals=IGBTVOverTempDiagEn
  Bus Selector1 : BusSelector  OutputSignals=IGBTVOverTempFltLevel,IGBTVOverTempPowerCoeff
  Diagnose : Subsystem
  EnableJudgement : Subsystem
  FaultLevelDeter : Subsystem
  Parameters : Subsystem
  PowerReductionCoeffDeter : Subsystem
  IGBTVOverTempFltInfo : Outport
  wires:
  Bus Selector/1 -> EnableJudgement/2(DiagEn)  "<IGBTVOverTempDiagEn>"
  Bus Selector1/2 -> PowerReductionCoeffDeter/2(PowerCoeff)  "<IGBTVOverTempPowerCoeff>"
  IGBTVTemp/1 -> Diagnose/2(IGBTVTemp), Parameters/1(IGBTVTemp)
  PowerReductionCoeffDeter/1(IGBTVOverTempPowerCoeffOut) -> Bus Creator/3  "IGBTVOverTempPowerCoeffOut"
  FaultLevelDeter/1(IGBTVOverTempFltLevelOut) -> PowerReductionCoeffDeter/1(IGBTVOverTempFltLevelOut), Bus Creator/2  "IGBTVOverTempFltLevelOut"
  Diagnose/1(IGBTVOverTempFlgOut) -> FaultLevelDeter/1(IGBTVOverTempFlgOut), Bus Creator/1  "IGBTVOverTempFlgOut"
  EnableJudgement/1(DiagEnOut) -> Diagnose/1(DiagEnOut)
  SysSelfCheckDownFlg/1 -> EnableJudgement/1(SysSelfCheckDownFlg)
  Parameters/1(Param) -> Bus Selector/1, Diagnose/3(Parameter), Bus Selector1/1
  Bus Creator/1 -> IGBTVOverTempFltInfo/1
  Bus Selector1/1 -> FaultLevelDeter/2(FaultLevel)  "<IGBTVOverTempFltLevel>"

== system FaultCheck/FaultDiagnose/IGBTTempDiag/IGBTWLowerTempDiag ==
  SysSelfCheckDownFlg : Inport
  IGBTWTemp : Inport  Port=2
  Bus Creator : BusCreator  Inputs=3
  Bus Selector : BusSelector  OutputSignals=IGBTWLowerTempDiagEn
  Bus Selector1 : BusSelector  OutputSignals=IGBTWLowerTempFltLevel,IGBTWLowerTempPowerCoeff
  Diagnose : Subsystem
  EnableJudgement : Subsystem
  FaultLevelDeter : Subsystem
  Parameters : Subsystem
  PowerReductionCoeffDeter : Subsystem
  IGBTWLowerTempFltInfo : Outport
  wires:
  Bus Selector1/1 -> FaultLevelDeter/2(FaultLevel)  "<IGBTWLowerTempFltLevel>"
  Bus Creator/1 -> IGBTWLowerTempFltInfo/1
  Parameters/1(Param) -> Bus Selector1/1, Diagnose/3(Parameter), Bus Selector/1
  SysSelfCheckDownFlg/1 -> EnableJudgement/1(SysSelfCheckDownFlg)
  EnableJudgement/1(DiagEnOut) -> Diagnose/1(DiagEnOut)
  Diagnose/1(IGBTWLowerTempFlgOut) -> Bus Creator/1, FaultLevelDeter/1(IGBTWLowerTempFlgOut)  "IGBTWLowerTempFlgOut"
  FaultLevelDeter/1(IGBTWLowerTempFltLevelOut) -> Bus Creator/2, PowerReductionCoeffDeter/1(IGBTWLowerTempFltLevelOut)  "IGBTWLowerTempFltLevelOut"
  PowerReductionCoeffDeter/1(IGBTWLowerTempPowerCoeffOut) -> Bus Creator/3  "IGBTWLowerTempPowerCoeffOut"
  IGBTWTemp/1 -> Diagnose/2(IGBTWTemp)
  Bus Selector1/2 -> PowerReductionCoeffDeter/2(PowerCoeff)  "<IGBTWLowerTempPowerCoeff>"
  Bus Selector/1 -> EnableJudgement/2(DiagEn)  "<IGBTWLowerTempDiagEn>"

== system FaultCheck/FaultDiagnose/IGBTTempDiag/IGBTWOverTempDiag ==
  SysSelfCheckDownFlg : Inport
  IGBTWTemp : Inport  Port=2
  Bus Creator : BusCreator  Inputs=3
  Bus Selector : BusSelector  OutputSignals=IGBTWOverTempDiagEn
  Bus Selector1 : BusSelector  OutputSignals=IGBTWOverTempFltLevel,IGBTWOverTempPowerCoeff
  Diagnose : Subsystem
  EnableJudgement : Subsystem
  FaultLevelDeter : Subsystem
  Parameters : Subsystem
  PowerReductionCoeffDeter : Subsystem
  IGBTWOverTempFltInfo : Outport
  wires:
  Bus Selector1/1 -> FaultLevelDeter/2(FaultLevel)  "<IGBTWOverTempFltLevel>"
  Bus Creator/1 -> IGBTWOverTempFltInfo/1
  Parameters/1(Param) -> Bus Selector1/1, Diagnose/3(Parameter), Bus Selector/1
  SysSelfCheckDownFlg/1 -> EnableJudgement/1(SysSelfCheckDownFlg)
  EnableJudgement/1(DiagEnOut) -> Diagnose/1(DiagEnOut)
  Diagnose/1(IGBTWOverTempFlgOut) -> Bus Creator/1, FaultLevelDeter/1(IGBTWOverTempFlgOut)  "IGBTWOverTempFlgOut"
  FaultLevelDeter/1(IGBTWOverTempFltLevelOut) -> Bus Creator/2, PowerReductionCoeffDeter/1(IGBTWOverTempFltLevelOut)  "IGBTWOverTempFltLevelOut"
  PowerReductionCoeffDeter/1(IGBTWOverTempPowerCoeffOut) -> Bus Creator/3  "IGBTWOverTempPowerCoeffOut"
  IGBTWTemp/1 -> Parameters/1(IGBTWTemp), Diagnose/2(IGBTWTemp)
  Bus Selector1/2 -> PowerReductionCoeffDeter/2(PowerCoeff)  "<IGBTWOverTempPowerCoeff>"
  Bus Selector/1 -> EnableJudgement/2(DiagEn)  "<IGBTWOverTempDiagEn>"

== system FaultCheck/FaultDiagnose/MotorSpdFltDiag/MotorOverSpdOneNegDiag ==
  SysSelfCheckDownFlg : Inport
  MotorSpd : Inport  Port=2
  Bus Creator : BusCreator  Inputs=3
  Bus Selector : BusSelector  OutputSignals=MotorOverSpdOneNegDiagEn
  Bus Selector1 : BusSelector  OutputSignals=MotorOverSpdOneNegFltLevel,MotorOverSpdOneNegPowerCoeff
  Diagnose : Subsystem
  EnableJudgement : Subsystem
  FaultLevelDeter : Subsystem
  Parameters : Subsystem
  PowerReductionCoeffDeter : Subsystem
  MotorOverSpdOneNegFltInfo : Outport
  wires:
  MotorSpd/1 -> Parameters/1(MotorSpd), Diagnose/2(MotorSpd)
  Bus Selector/1 -> EnableJudgement/2(DiagEn)  "<MotorOverSpdOneNegDiagEn>"
  Bus Selector1/2 -> PowerReductionCoeffDeter/2(PowerCoeff)  "<MotorOverSpdOneNegPowerCoeff>"
  Bus Creator/1 -> MotorOverSpdOneNegFltInfo/1
  EnableJudgement/1(DiagEnOut) -> Diagnose/1(DiagEnOut)
  FaultLevelDeter/1(MotorOverSpdOneNegFltLevelOut) -> Bus Creator/2, PowerReductionCoeffDeter/1(MotorOverSpdOneNegFltLevelOut)  "MotorOverSpdOneNegFltLevelOut"
  Diagnose/1(MotorOverSpdOneNegFlgOut) -> Bus Creator/1, FaultLevelDeter/1(MotorOverSpdOneNegFlgOut)  "MotorOverSpdOneNegFlgOut"
  Bus Selector1/1 -> FaultLevelDeter/2(FaultLevel)  "<MotorOverSpdOneNegFltLevel>"
  Parameters/1(Param) -> Bus Selector1/1, Diagnose/3(Parameter), Bus Selector/1
  SysSelfCheckDownFlg/1 -> EnableJudgement/1(SysSelfCheckDownFlg)
  PowerReductionCoeffDeter/1(MotorOverSpdOneNegPowerCoeffOut) -> Bus Creator/3  "MotorOverSpdOneNegPowerCoeffOut"

== system FaultCheck/FaultDiagnose/MotorSpdFltDiag/MotorOverSpdOnePosDiag ==
  SysSelfCheckDownFlg : Inport
  MotorSpd : Inport  Port=2
  Bus Creator : BusCreator  Inputs=3
  Bus Selector : BusSelector  OutputSignals=MotorOverSpdOnePosDiagEn
  Bus Selector1 : BusSelector  OutputSignals=MotorOverSpdOnePosFltLevel,MotorOverSpdOnePosPowerCoeff
  Diagnose : Subsystem
  EnableJudgement : Subsystem
  FaultLevelDeter : Subsystem
  Parameters : Subsystem
  PowerReductionCoeffDeter : Subsystem
  MotorOverSpdOnePosFltInfo : Outport
  wires:
  Bus Selector1/1 -> FaultLevelDeter/2(FaultLevel)  "<MotorOverSpdOnePosFltLevel>"
  Bus Creator/1 -> MotorOverSpdOnePosFltInfo/1
  Parameters/1(Param) -> Bus Selector1/1, Diagnose/3(Parameter), Bus Selector/1
  SysSelfCheckDownFlg/1 -> EnableJudgement/1(SysSelfCheckDownFlg)
  EnableJudgement/1(DiagEnOut) -> Diagnose/1(DiagEnOut)
  Diagnose/1(MotorOverSpdOnePosFlgOut) -> Bus Creator/1, FaultLevelDeter/1(MotorOverSpdOnePosFlgOut)  "MotorOverSpdOnePosFlgOut"
  FaultLevelDeter/1(MotorOverSpdOnePosFltLevelOut) -> Bus Creator/2, PowerReductionCoeffDeter/1(MotorOverSpdOnePosFltLevelOut)  "MotorOverSpdOnePosFltLevelOut"
  PowerReductionCoeffDeter/1(MotorOverSpdOnePosPowerCoeffOut) -> Bus Creator/3  "MotorOverSpdOnePosPowerCoeffOut"
  MotorSpd/1 -> Parameters/1(MotorSpd), Diagnose/2(MotorSpd)
  Bus Selector1/2 -> PowerReductionCoeffDeter/2(PowerCoeff)  "<MotorOverSpdOnePosPowerCoeff>"
  Bus Selector/1 -> EnableJudgement/2(DiagEn)  "<MotorOverSpdOnePosDiagEn>"

== system FaultCheck/FaultDiagnose/MotorSpdFltDiag/MotorOverSpdTwoNegDiag ==
  SysSelfCheckDownFlg : Inport
  MotorSpd : Inport  Port=2
  Bus Creator : BusCreator  Inputs=3
  Bus Selector : BusSelector  OutputSignals=MotorOverSpdTwoNegDiagEn
  Bus Selector1 : BusSelector  OutputSignals=MotorOverSpdTwoNegFltLevel,MotorOverSpdTwoNegPowerCoeff
  Diagnose : Subsystem
  EnableJudgement : Subsystem
  FaultLevelDeter : Subsystem
  Parameters : Subsystem
  PowerReductionCoeffDeter : Subsystem
  MotorOverSpdTwoNegFltInfo : Outport
  wires:
  PowerReductionCoeffDeter/1(MotorOverSpdTwoNegPowerCoeffOut) -> Bus Creator/3  "MotorOverSpdTwoNegPowerCoeffOut"
  SysSelfCheckDownFlg/1 -> EnableJudgement/1(SysSelfCheckDownFlg)
  Parameters/1(Param) -> Bus Selector/1, Diagnose/3(Parameter), Bus Selector1/1
  Bus Selector1/1 -> FaultLevelDeter/2(FaultLevel)  "<MotorOverSpdTwoNegFltLevel>"
  Diagnose/1(MotorOverSpdTwoNegFlgOut) -> FaultLevelDeter/1(MotorOverSpdTwoNegFlgOut), Bus Creator/1  "MotorOverSpdTwoNegFlgOut"
  FaultLevelDeter/1(MotorOverSpdTwoNegFltLevelOut) -> PowerReductionCoeffDeter/1(MotorOverSpdTwoNegFltLevelOut), Bus Creator/2  "MotorOverSpdTwoNegFltLevelOut"
  EnableJudgement/1(DiagEnOut) -> Diagnose/1(DiagEnOut)
  Bus Creator/1 -> MotorOverSpdTwoNegFltInfo/1
  Bus Selector1/2 -> PowerReductionCoeffDeter/2(PowerCoeff)  "<MotorOverSpdTwoNegPowerCoeff>"
  Bus Selector/1 -> EnableJudgement/2(DiagEn)  "<MotorOverSpdTwoNegDiagEn>"
  MotorSpd/1 -> Diagnose/2(MotorSpd)

== system FaultCheck/FaultDiagnose/MotorSpdFltDiag/MotorOverSpdTwoPosDiag ==
  SysSelfCheckDownFlg : Inport
  MotorSpd : Inport  Port=2
  Bus Creator : BusCreator  Inputs=3
  Bus Selector : BusSelector  OutputSignals=MotorOverSpdTwoPosDiagEn
  Bus Selector1 : BusSelector  OutputSignals=MotorOverSpdTwoPosFltLevel,MotorOverSpdTwoPosPowerCoeff
  Diagnose : Subsystem
  EnableJudgement : Subsystem
  FaultLevelDeter : Subsystem
  Parameters : Subsystem
  PowerReductionCoeffDeter : Subsystem
  MotorOverSpdTwoPosFltInfo : Outport
  wires:
  Bus Selector/1 -> EnableJudgement/2(DiagEn)  "<MotorOverSpdTwoPosDiagEn>"
  Bus Selector1/2 -> PowerReductionCoeffDeter/2(PowerCoeff)  "<MotorOverSpdTwoPosPowerCoeff>"
  MotorSpd/1 -> Diagnose/2(MotorSpd)
  PowerReductionCoeffDeter/1(MotorOverSpdTwoPosPowerCoeffOut) -> Bus Creator/3  "MotorOverSpdTwoPosPowerCoeffOut"
  FaultLevelDeter/1(MotorOverSpdTwoPosFltLevelOut) -> PowerReductionCoeffDeter/1(MotorOverSpdTwoPosFltLevelOut), Bus Creator/2  "MotorOverSpdTwoPosFltLevelOut"
  Diagnose/1(MotorOverSpdTwoPosFlgOut) -> FaultLevelDeter/1(MotorOverSpdTwoPosFlgOut), Bus Creator/1  "MotorOverSpdTwoPosFlgOut"
  EnableJudgement/1(DiagEnOut) -> Diagnose/1(DiagEnOut)
  SysSelfCheckDownFlg/1 -> EnableJudgement/1(SysSelfCheckDownFlg)
  Parameters/1(Param) -> Bus Selector/1, Diagnose/3(Parameter), Bus Selector1/1
  Bus Creator/1 -> MotorOverSpdTwoPosFltInfo/1
  Bus Selector1/1 -> FaultLevelDeter/2(FaultLevel)  "<MotorOverSpdTwoPosFltLevel>"

== system FaultCheck/FaultDiagnose/MotorTempDiag/MotorLowerTempDiag ==
  SysSelfCheckDownFlg : Inport
  MotorTemp : Inport  Port=2
  Bus Creator : BusCreator  Inputs=3
  Bus Selector : BusSelector  OutputSignals=MotorLowerTempDiagEn
  Bus Selector1 : BusSelector  OutputSignals=MotorLowerTempFltLevel,MotorLowerTempPowerCoeff
  Diagnose : Subsystem
  EnableJudgement : Subsystem
  FaultLevelDeter : Subsystem
  Parameters : Subsystem
  PowerReductionCoeffDeter : Subsystem
  MotorLowerTempFltInfo : Outport
  wires:
  Bus Selector/1 -> EnableJudgement/2(DiagEn)  "<MotorLowerTempDiagEn>"
  Bus Selector1/2 -> PowerReductionCoeffDeter/2(PowerCoeff)  "<MotorLowerTempPowerCoeff>"
  MotorTemp/1 -> Diagnose/2(MotorTemp)
  PowerReductionCoeffDeter/1(MotorLowerTempPowerCoeffOut) -> Bus Creator/3  "MotorLowerTempPowerCoeffOut"
  FaultLevelDeter/1(MotorLowerTempFltLevelOut) -> PowerReductionCoeffDeter/1(MotorLowerTempFltLevelOut), Bus Creator/2  "MotorLowerTempFltLevelOut"
  Diagnose/1(MotorLowerTempFlgOut) -> FaultLevelDeter/1(MotorLowerTempFlgOut), Bus Creator/1  "MotorLowerTempFlgOut"
  EnableJudgement/1(DiagEnOut) -> Diagnose/1(DiagEnOut)
  SysSelfCheckDownFlg/1 -> EnableJudgement/1(SysSelfCheckDownFlg)
  Parameters/1(Param) -> Bus Selector/1, Diagnose/3(Parameter), Bus Selector1/1
  Bus Creator/1 -> MotorLowerTempFltInfo/1
  Bus Selector1/1 -> FaultLevelDeter/2(FaultLevel)  "<MotorLowerTempFltLevel>"

== system FaultCheck/FaultDiagnose/MotorTempDiag/MotorOverTempDiag ==
  SysSelfCheckDownFlg : Inport
  MotorTemp : Inport  Port=2
  Bus Creator : BusCreator  Inputs=3
  Bus Selector : BusSelector  OutputSignals=MotorOverTempDiagEn
  Bus Selector1 : BusSelector  OutputSignals=MotorOverTempFltLevel,MotorOverTempPowerCoeff
  Diagnose : Subsystem
  EnableJudgement : Subsystem
  FaultLevelDeter : Subsystem
  Parameters : Subsystem
  PowerReductionCoeffDeter : Subsystem
  MotorOverTempFltInfo : Outport
  wires:
  Bus Selector1/1 -> FaultLevelDeter/2(FaultLevel)  "<MotorOverTempFltLevel>"
  Bus Creator/1 -> MotorOverTempFltInfo/1
  Parameters/1(Param) -> Bus Selector1/1, Diagnose/3(Parameter), Bus Selector/1
  SysSelfCheckDownFlg/1 -> EnableJudgement/1(SysSelfCheckDownFlg)
  EnableJudgement/1(DiagEnOut) -> Diagnose/1(DiagEnOut)
  Diagnose/1(MotorOverTempFlgOut) -> Bus Creator/1, FaultLevelDeter/1(MotorOverTempFlgOut)  "MotorOverTempFlgOut"
  FaultLevelDeter/1(MotorOverTempFltLevelOut) -> Bus Creator/2, PowerReductionCoeffDeter/1(MotorOverTempFltLevelOut)  "MotorOverTempFltLevelOut"
  PowerReductionCoeffDeter/1(MotorOverTempPowerCoeffOut) -> Bus Creator/3  "MotorOverTempPowerCoeffOut"
  MotorTemp/1 -> Parameters/1(MotorTemp), Diagnose/2(MotorTemp)
  Bus Selector1/2 -> PowerReductionCoeffDeter/2(PowerCoeff)  "<MotorOverTempPowerCoeff>"
  Bus Selector/1 -> EnableJudgement/2(DiagEn)  "<MotorOverTempDiagEn>"

== system FaultCheck/FaultDiagnose/PCBTempDiag/PCBLowerTempDiag ==
  SysSelfCheckDownFlg : Inport
  PCBTemp : Inport  Port=2
  Bus Creator : BusCreator  Inputs=3
  Bus Selector : BusSelector  OutputSignals=PCBLowerTempDiagEn
  Bus Selector1 : BusSelector  OutputSignals=PCBLowerTempFltLevel,PCBLowerTempPowerCoeff
  Diagnose : Subsystem
  EnableJudgement : Subsystem
  FaultLevelDeter : Subsystem
  Parameters : Subsystem
  PowerReductionCoeffDeter : Subsystem
  PCBLowerTempFltInfo : Outport
  wires:
  Bus Selector/1 -> EnableJudgement/2(DiagEn)  "<PCBLowerTempDiagEn>"
  Bus Selector1/2 -> PowerReductionCoeffDeter/2(PowerCoeff)  "<PCBLowerTempPowerCoeff>"
  PCBTemp/1 -> Diagnose/2(PCBTemp)
  PowerReductionCoeffDeter/1(PCBLowerTempPowerCoeffOut) -> Bus Creator/3  "PCBLowerTempPowerCoeffOut"
  FaultLevelDeter/1(PCBLowerTempFltLevelOut) -> PowerReductionCoeffDeter/1(PCBLowerTempFltLevelOut), Bus Creator/2  "PCBLowerTempFltLevelOut"
  Diagnose/1(PCBLowerTempFlgOut) -> FaultLevelDeter/1(PCBLowerTempFlgOut), Bus Creator/1  "PCBLowerTempFlgOut"
  EnableJudgement/1(DiagEnOut) -> Diagnose/1(DiagEnOut)
  SysSelfCheckDownFlg/1 -> EnableJudgement/1(SysSelfCheckDownFlg)
  Parameters/1(Param) -> Bus Selector/1, Diagnose/3(Parameter), Bus Selector1/1
  Bus Creator/1 -> PCBLowerTempFltInfo/1
  Bus Selector1/1 -> FaultLevelDeter/2(FaultLevel)  "<PCBLowerTempFltLevel>"

== system FaultCheck/FaultDiagnose/PCBTempDiag/PCBOverTempDiag ==
  SysSelfCheckDownFlg : Inport
  PCBTemp : Inport  Port=2
  Bus Creator : BusCreator  Inputs=3
  Bus Selector : BusSelector  OutputSignals=PCBOverTempDiagEn
  Bus Selector1 : BusSelector  OutputSignals=PCBOverTempFltLevel,PCBOverTempPowerCoeff
  Diagnose : Subsystem
  EnableJudgement : Subsystem
  FaultLevelDeter : Subsystem
  Parameters : Subsystem
  PowerReductionCoeffDeter : Subsystem
  PCBOverTempFltInfo : Outport
  wires:
  Bus Selector1/1 -> FaultLevelDeter/2(FaultLevel)  "<PCBOverTempFltLevel>"
  Bus Creator/1 -> PCBOverTempFltInfo/1
  Parameters/1(Param) -> Bus Selector1/1, Diagnose/3(Parameter), Bus Selector/1
  SysSelfCheckDownFlg/1 -> EnableJudgement/1(SysSelfCheckDownFlg)
  EnableJudgement/1(DiagEnOut) -> Diagnose/1(DiagEnOut)
  Diagnose/1(PCBOverTempFlgOut) -> Bus Creator/1, FaultLevelDeter/1(PCBOverTempFlgOut)  "PCBOverTempFlgOut"
  FaultLevelDeter/1(PCBOverTempFltLevelOut) -> Bus Creator/2, PowerReductionCoeffDeter/1(PCBOverTempFltLevelOut)  "PCBOverTempFltLevelOut"
  PowerReductionCoeffDeter/1(PCBOverTempPowerCoeffOut) -> Bus Creator/3  "PCBOverTempPowerCoeffOut"
  PCBTemp/1 -> Parameters/1(PCBTemp), Diagnose/2(PCBTemp)
  Bus Selector1/2 -> PowerReductionCoeffDeter/2(PowerCoeff)  "<PCBOverTempPowerCoeff>"
  Bus Selector/1 -> EnableJudgement/2(DiagEn)  "<PCBOverTempDiagEn>"

== system FaultCheck/FaultDiagnose/PhaseCurrDiag/Flt_IuOverCurrDiag ==
  SysSelfCheckDownFlg : Inport
  UPhaseCurr_A : Inport  Port=2
  Bus Creator : BusCreator  Inputs=3
  Bus Selector : BusSelector  OutputSignals=IuOCPowerCoeff
  Diagnose : Subsystem
  FaultLevelDeter : Subsystem
  Parameters : Subsystem
  PowerReductionCoeffDeter : Subsystem
  IuOverCurrFltInfoOut : Outport
  wires:
  UPhaseCurr_A/1 -> Diagnose/3(UPhaseCurr_A)
  SysSelfCheckDownFlg/1 -> Diagnose/1(SysSelfCheckDownFlg)
  Parameters/1(IuOCParam) -> FaultLevelDeter/2(IuOCParam), Bus Selector/1, Diagnose/2(IuOCParam)
  Diagnose/1(IuOCFltFlg) -> FaultLevelDeter/1(IuOCFltFlg), Bus Creator/1
  Bus Creator/1 -> IuOverCurrFltInfoOut/1
  FaultLevelDeter/1(IuOCFltLevelOut) -> PowerReductionCoeffDeter/1(IuOCFltLevelOut), Bus Creator/2
  PowerReductionCoeffDeter/1(IuOCPowerCoeff) -> Bus Creator/3
  Bus Selector/1 -> PowerReductionCoeffDeter/2(PowerCoeff)  "<IuOCPowerCoeff>"

== system FaultCheck/FaultDiagnose/PhaseCurrDiag/Flt_IvOverCurrDiag ==
  note: TODO：
      | 1：故障码
  SysSelfCheckDownFlg : Inport
  VPhaseCurr_A : Inport  Port=2
  Bus Creator : BusCreator  Inputs=3
  Bus Selector : BusSelector  OutputSignals=IvOCPowerCoeff
  Diagnose : Subsystem
  FaultLevelDeter : Subsystem
  Parameters : Subsystem
  PowerReductionCoeffDeter : Subsystem
  IvOverCurrFltInfoOut : Outport
  wires:
  Bus Selector/1 -> PowerReductionCoeffDeter/2(PowerCoeff)  "<IvOCPowerCoeff>"
  PowerReductionCoeffDeter/1(IvOCPowerCoeff) -> Bus Creator/3
  FaultLevelDeter/1(IvOCFltLevelOut) -> Bus Creator/2, PowerReductionCoeffDeter/1(IvOCFltLevelOut)
  Bus Creator/1 -> IvOverCurrFltInfoOut/1
  Diagnose/1(IvOCFltFlg) -> Bus Creator/1, FaultLevelDeter/1(IvOCFltFlg)
  Parameters/1(IvOCParam) -> Diagnose/2(IvOCParam), Bus Selector/1, FaultLevelDeter/2(IvOCParam)
  SysSelfCheckDownFlg/1 -> Diagnose/1(SysSelfCheckDownFlg)
  VPhaseCurr_A/1 -> Diagnose/3(VPhaseCurr_A)

== system FaultCheck/FaultDiagnose/PhaseCurrDiag/Flt_IwOverCurrDiag ==
  note: TODO：
      | 1：故障码
  SysSelfCheckDownFlg : Inport
  WPhaseCurr_A : Inport  Port=2
  Bus Creator : BusCreator  Inputs=3
  Bus Selector : BusSelector  OutputSignals=IwOCPowerCoeff
  Diagnose : Subsystem
  FaultLevelDeter : Subsystem
  Parameters : Subsystem
  PowerReductionCoeffDeter : Subsystem
  IwOverCurrFltInfoOut : Outport
  wires:
  WPhaseCurr_A/1 -> Diagnose/3(VPhaseCurr_A)
  SysSelfCheckDownFlg/1 -> Diagnose/1(SysSelfCheckDownFlg)
  Parameters/1(IwOCParam) -> FaultLevelDeter/2(IwOCParam), Bus Selector/1, Diagnose/2(IwOCParam)
  Diagnose/1(IwOCFltFlg) -> FaultLevelDeter/1(IwOCFltFlg), Bus Creator/1
  Bus Creator/1 -> IwOverCurrFltInfoOut/1
  FaultLevelDeter/1(IwOCFltLevelOut) -> PowerReductionCoeffDeter/1(IwOCFltLevelOut), Bus Creator/2
  PowerReductionCoeffDeter/1(IwOCPowerCoeff) -> Bus Creator/3
  Bus Selector/1 -> PowerReductionCoeffDeter/2(PowerCoeff)  "<IwOCPowerCoeff>"

== system FaultCheck/FaultDiagnose/UdcLowerOneDiag/Diagnose ==
  DiagEnOut : Inport
  Udc : Inport  Port=2
  Parameter : Inport  Port=3
  Disable : Subsystem  TreatAsAtomicUnit=on
  If : If  IfExpression=u1 == 0
  Merge : Merge
  NormalDiag : Subsystem  TreatAsAtomicUnit=on
  UdcLowerOneFlgOut : Outport
  wires:
  DiagEnOut/1 -> If/1
  If/1 -> Disable/Action
  If/2 -> NormalDiag/Action
  Udc/1 -> NormalDiag/1(Udc)
  Parameter/1 -> NormalDiag/2(Parameter)
  Disable/1(UdcLowerOneFltDeb) -> Merge/1
  NormalDiag/1(UdcLowerOneFltDeb) -> Merge/2
  Merge/1 -> UdcLowerOneFlgOut/1  "M_Flt_UdcLowerOneFlgOut_b"

== system FaultCheck/FaultDiagnose/UdcLowerOneDiag/EnableJudgement ==
  SysSelfCheckDownFlg : Inport
  DiagEn : Inport  Port=2
  Constant : Constant  Value=true
  Logical Operator : Logic  AllPortsSameDT=off  OutDataTypeStr=boolean
  Logical Operator1 : Logic  AllPortsSameDT=off  OutDataTypeStr=boolean
  Logical Operator2 : Logic  AllPortsSameDT=off  OutDataTypeStr=boolean
  DiagEnOut : Outport
  wires:
  Logical Operator2/1 -> DiagEnOut/1  "M_Flt_UdcLowerOneDiagEn_b"
  Logical Operator/1 -> Logical Operator2/1
  SysSelfCheckDownFlg/1 -> Logical Operator/2
  DiagEn/1 -> Logical Operator1/2
  Constant/1 -> Logical Operator/1, Logical Operator1/1
  Logical Operator1/1 -> Logical Operator2/2

== system FaultCheck/FaultDiagnose/UdcLowerOneDiag/FaultLevelDeter ==
  UdcLowerOneFlgOut : Inport
  FaultLevel : Inport  Port=2
  If : If  IfExpression=u1 == 0
  LowerOne : Subsystem  TreatAsAtomicUnit=on
  Merge : Merge
  Normal : Subsystem  TreatAsAtomicUnit=on
  UdcLowerOneFltLevelOut : Outport
  wires:
  UdcLowerOneFlgOut/1 -> If/1
  If/1 -> Normal/Action
  If/2 -> LowerOne/Action
  Normal/1(UdcLowerOneFltLevel) -> Merge/1
  LowerOne/1(UdcLowerOneFltLevel) -> Merge/2
  Merge/1 -> UdcLowerOneFltLevelOut/1  "M_Flt_UdcLowerOneFltLevelOut_u8"
  FaultLevel/1 -> LowerOne/1(FaultLevel)

== system FaultCheck/FaultDiagnose/UdcLowerOneDiag/Parameters ==
  Udc : Inport
  1-D Lookup Table1 : Lookup_n-D  NumberOfTableDimensions=1  BreakpointsForDimension1=[-5:5]  BreakpointsForDimension1DataTypeStr=Inherit: Inherit from 'Breakpoint data'  IndexSearchMethod=Linear search  Table=tanh([-5:5])  TableDataTypeStr=Inherit: Inherit from 'Table data'  ExtrapMethod=Clip  UseLastTableValue=on  InternalRulePriority=Speed  OutDataTypeStr=single  RndMeth=Simplest
  Bus Creator : BusCreator  Inputs=8
  Constant : Constant  Value=C_Flt_UdcLowerOneTrigTh_s32
  Constant1 : Constant  Value=C_Flt_UdcLowerOneRecTh_s32
  Constant10 : Constant  Value=C_Flt_UdcLowerOneRecoveryTh_u16
  Constant11 : Constant  Value=C_Flt_LevelTwo_u8
  Constant7 : Constant  Value=C_Flt_UdcLowerOneDiagEn_b
  Constant8 : Constant  Value=C_Flt_UdcLowerOneErrCode_u16
  Constant9 : Constant  Value=C_Flt_UdcLowerOneConfirmTh_u16
  Param : Outport
  wires:
  Bus Creator/1 -> Param/1
  Udc/1 -> 1-D Lookup Table1/1
  Constant/1 -> Bus Creator/1  "UdcLowerOneTrigTh"
  Constant7/1 -> Bus Creator/3  "UdcLowerOneDiagEn"
  Constant8/1 -> Bus Creator/4  "UdcLowerOneErrCode"
  Constant9/1 -> Bus Creator/5  "UdcLowerOneConfirmTh"
  Constant10/1 -> Bus Creator/6  "UdcLowerOneRecoveryTh"
  Constant11/1 -> Bus Creator/7  "UdcLowerOneFltLevel"
  1-D Lookup Table1/1 -> Bus Creator/8  "UdcLowerOnePowerCoeff"
  Constant1/1 -> Bus Creator/2  "UdcLowerOneRecTh"

== system FaultCheck/FaultDiagnose/UdcLowerOneDiag/PowerReductionCoeffDeter ==
  UdcLowerOneFltLevelOut : Inport
  PowerCoeff : Inport  Port=2
  If : If  IfExpression=u1 < 2  ElseIfExpressions=u1 == 2
  If Action Subsystem : Subsystem  TreatAsAtomicUnit=on
  If Action Subsystem1 : Subsystem  TreatAsAtomicUnit=on
  If Action Subsystem2 : Subsystem  TreatAsAtomicUnit=on
  Merge : Merge  Inputs=3
  UdcLowerOnePowerCoeffOut : Outport
  wires:
  UdcLowerOneFltLevelOut/1 -> If/1
  If/1 -> If Action Subsystem/Action
  If/2 -> If Action Subsystem1/Action
  If/3 -> If Action Subsystem2/Action
  PowerCoeff/1 -> If Action Subsystem1/1(PowerCoeff)
  If Action Subsystem/1(Coeff) -> Merge/1
  If Action Subsystem1/1(Coeff) -> Merge/2
  If Action Subsystem2/1(Coeff) -> Merge/3
  Merge/1 -> UdcLowerOnePowerCoeffOut/1  "M_Flt_UdcLowerOnePowerCoeffOut_s32"

== system FaultCheck/FaultDiagnose/UdcLowerTwoDiag/Diagnose ==
  DiagEnOut : Inport
  Udc : Inport  Port=2
  Parameter : Inport  Port=3
  Disable : Subsystem  TreatAsAtomicUnit=on
  If : If  IfExpression=u1 == 0
  Merge : Merge
  NormalDiag : Subsystem  TreatAsAtomicUnit=on
  UdcLowerTwoFlgOut : Outport
  wires:
  DiagEnOut/1 -> If/1
  If/1 -> Disable/Action
  If/2 -> NormalDiag/Action
  Udc/1 -> NormalDiag/1(Udc)
  Parameter/1 -> NormalDiag/2(Parameter)
  Disable/1(UdcLowerTwoFltDeb) -> Merge/1
  NormalDiag/1(UdcLowerTwoFltDeb) -> Merge/2
  Merge/1 -> UdcLowerTwoFlgOut/1  "M_Flt_UdcLowerTwoFlgOut_b"

== system FaultCheck/FaultDiagnose/UdcLowerTwoDiag/EnableJudgement ==
  SysSelfCheckDownFlg : Inport
  DiagEn : Inport  Port=2
  Constant : Constant  Value=true
  Logical Operator : Logic  AllPortsSameDT=off  OutDataTypeStr=boolean
  Logical Operator1 : Logic  AllPortsSameDT=off  OutDataTypeStr=boolean
  Logical Operator2 : Logic  AllPortsSameDT=off  OutDataTypeStr=boolean
  DiagEnOut : Outport
  wires:
  Logical Operator2/1 -> DiagEnOut/1  "M_Flt_UdcLowerTwoDiagEn_b"
  Logical Operator/1 -> Logical Operator2/1
  SysSelfCheckDownFlg/1 -> Logical Operator/2
  DiagEn/1 -> Logical Operator1/2
  Constant/1 -> Logical Operator/1, Logical Operator1/1
  Logical Operator1/1 -> Logical Operator2/2

== system FaultCheck/FaultDiagnose/UdcLowerTwoDiag/FaultLevelDeter ==
  UdcLowerTwoFlgOut : Inport
  FaultLevel : Inport  Port=2
  If : If  IfExpression=u1 == 0
  LowerTwo : Subsystem  TreatAsAtomicUnit=on
  Merge : Merge
  Normal : Subsystem  TreatAsAtomicUnit=on
  UdcLowerTwoFltLevelOut : Outport
  wires:
  UdcLowerTwoFlgOut/1 -> If/1
  If/1 -> Normal/Action
  If/2 -> LowerTwo/Action
  Normal/1(UdcLowerTwoFltLevel) -> Merge/1
  LowerTwo/1(UdcLowerTwoFltLevel) -> Merge/2
  Merge/1 -> UdcLowerTwoFltLevelOut/1  "M_Flt_UdcLowerTwoFltLevelOut_u8"
  FaultLevel/1 -> LowerTwo/1(FaultLevel)

== system FaultCheck/FaultDiagnose/UdcLowerTwoDiag/Parameters ==
  Bus Creator : BusCreator  Inputs=8
  Constant : Constant  Value=C_Flt_UdcLowerTwoTrigTh_s32
  Constant1 : Constant  Value=C_Flt_PowerCoeffZero_s32
  Constant10 : Constant  Value=C_Flt_UdcLowerTwoRecoveryTh_u16
  Constant11 : Constant  Value=C_Flt_LevelThree_u8
  Constant2 : Constant  Value=C_Flt_UdcLowerTwoRecTh_s32
  Constant7 : Constant  Value=C_Flt_UdcLowerTwoDiagEn_b
  Constant8 : Constant  Value=C_Flt_UdcLowerTwoErrCode_u16
  Constant9 : Constant  Value=C_Flt_UdcLowerTwoConfirmTh_u16
  Param : Outport
  wires:
  Bus Creator/1 -> Param/1
  Constant/1 -> Bus Creator/1  "UdcLowerTwoTrigTh"
  Constant7/1 -> Bus Creator/3  "UdcLowerTwoDiagEn"
  Constant8/1 -> Bus Creator/4  "UdcLowerTwoErrCode"
  Constant9/1 -> Bus Creator/5  "UdcLowerTwoConfirmTh"
  Constant10/1 -> Bus Creator/6  "UdcLowerTwoRecoveryTh"
  Constant11/1 -> Bus Creator/7  "UdcLowerTwoFltLevel"
  Constant1/1 -> Bus Creator/8  "UdcLowerTwoPowerCoeff"
  Constant2/1 -> Bus Creator/2  "UdcLowerTwoRecTh"

== system FaultCheck/FaultDiagnose/UdcLowerTwoDiag/PowerReductionCoeffDeter ==
  UdcLowerTwoFltLevelOut : Inport
  PowerCoeff : Inport  Port=2
  If : If  IfExpression=u1 < 2  ElseIfExpressions=u1 == 2
  If Action Subsystem : Subsystem  TreatAsAtomicUnit=on
  If Action Subsystem1 : Subsystem  TreatAsAtomicUnit=on
  If Action Subsystem2 : Subsystem  TreatAsAtomicUnit=on
  Merge : Merge  Inputs=3
  UdcLowerTwoPowerCoeffOut : Outport
  wires:
  UdcLowerTwoFltLevelOut/1 -> If/1
  If/1 -> If Action Subsystem/Action
  If/2 -> If Action Subsystem1/Action
  If/3 -> If Action Subsystem2/Action
  PowerCoeff/1 -> If Action Subsystem1/1(PowerCoeff)
  If Action Subsystem/1(Coeff) -> Merge/1
  If Action Subsystem1/1(Coeff) -> Merge/2
  If Action Subsystem2/1(Coeff) -> Merge/3
  Merge/1 -> UdcLowerTwoPowerCoeffOut/1  "M_Flt_UdcLowerTwoPowerCoeffOut_s32"
